simulink model "RLC"  (R2019b)
settings: Solver=VariableStepAuto  StartTime=0.0  StopTime=10.0  MaxStep=1e-4  RelTol=1e-8
values from neighbouring files (symbols this model uses):
  C = 1    [RLC_S.m]
  IC_int = -VC_int/R-IL_int    (= -6)    [RLC_S.m]
  L = 0.3    [Pendulumn_1.m]    (also in RLC_S.m = 1)
  R = 1    [RLC_S.m]
  VC_int = 5    [RLC_S.m]
undefined symbols (not defined in the file or in its folder): Vin
settings Model: Creator=xiadh  LastModifiedBy=xiadh

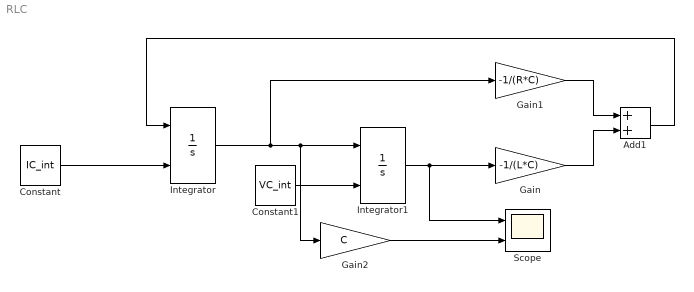
== system RLC ==
  Add1 : Sum
  Constant : Constant  Value=IC_int
  Constant1 : Constant  Value=VC_int
  Gain : Gain  Gain=-1/(L*C)
  Gain1 : Gain  Gain=-1/(R*C)
  Gain2 : Gain  Gain=C
  Integrator : Integrator  InitialConditionSource=external  UpperSaturationLimit=0  LowerSaturationLimit=-Vin/R
  Integrator1 : Integrator  InitialConditionSource=external  UpperSaturationLimit=Vin  LowerSaturationLimit=0
  Scope : Scope  NumInputPorts=2
  wires:
  Integrator/1 -> Gain1/1, Gain2/1, Integrator1/1
  Integrator1/1 -> Scope/1, Gain/1
  Gain1/1 -> Add1/1
  Gain/1 -> Add1/2
  Add1/1 -> Integrator/1
  Constant/1 -> Integrator/2
  Constant1/1 -> Integrator1/2
  Gain2/1 -> Scope/2
